simulink model "wiper_system"  (R2022b)
settings: Solver=VariableStepAuto  StartTime=0.0  StopTime=10  MaxStep=1e-3  RelTol=1e-3
undefined symbols (not defined in the file or in its folder): wiper_mode
settings Model: Creator=Dell  LastModifiedBy=Dell
settings DataIOCC: ExternalInput=[t, in1,in2]  SaveFormat=Array
settings DebuggingCC: ParameterPrecisionLossMsg=none

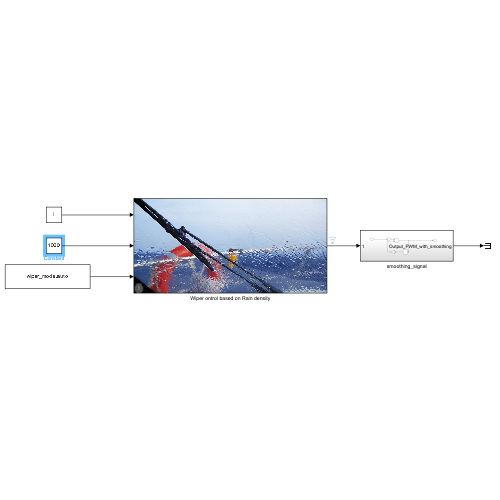
[thumbnail: Simulink's stored preview of the top-level diagram]
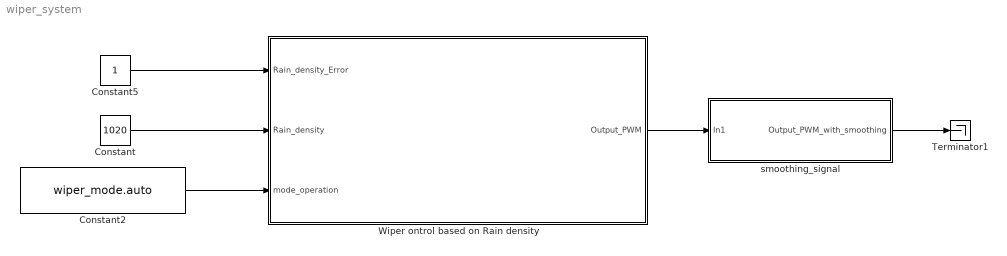
== system wiper_system ==
  Constant : Constant  Value=1020
  Constant2 : Constant  Value=wiper_mode.auto  OutDataTypeStr=Enum: wiper_mode
  Constant5 : Constant
  Terminator1 : Terminator
  Wiper ontrol based on Rain density : Subsystem
      mask Display: image('wiper.jpg');
  smoothing_signal : Subsystem
  wires:
  Constant5/1 -> Wiper ontrol based on Rain density/1(Rain_density_Error)
  Constant/1 -> Wiper ontrol based on Rain density/2(Rain_density)
  Constant2/1 -> Wiper ontrol based on Rain density/3(mode_operation)
  Wiper ontrol based on Rain density/1(Output_PWM) -> smoothing_signal/1(In1)
  smoothing_signal/1(Output_PWM_with_smoothing) -> Terminator1/1

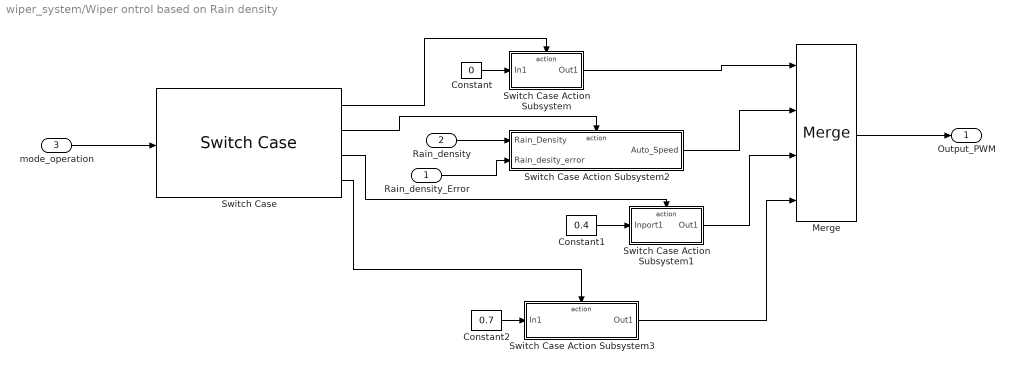
== system wiper_system/Wiper ontrol based on Rain density ==
  Rain_density_Error : Inport
  Rain_density : Inport  Port=2
  mode_operation : Inport  Port=3
  Constant : Constant  Value=0
  Constant1 : Constant  Value=0.4
  Constant2 : Constant  Value=0.7
  Merge : Merge  Inputs=4
  Switch Case : SwitchCase  CaseConditions=[wiper_mode.off,wiper_mode.auto,wiper_mode.low_speed,wiper_mode.high_speed]  ShowDefaultCase=off
  Switch Case Action Subsystem : Subsystem  TreatAsAtomicUnit=on
  Switch Case Action Subsystem1 : Subsystem  TreatAsAtomicUnit=on
  Switch Case Action Subsystem2 : Subsystem  TreatAsAtomicUnit=on
  Switch Case Action Subsystem3 : Subsystem  TreatAsAtomicUnit=on
  Output_PWM : Outport
  wires:
  Switch Case/1 -> Switch Case Action Subsystem/Action
  Switch Case/2 -> Switch Case Action Subsystem2/Action
  Switch Case/3 -> Switch Case Action Subsystem1/Action
  Switch Case/4 -> Switch Case Action Subsystem3/Action
  Constant2/1 -> Switch Case Action Subsystem3/1(In1)
  Constant1/1 -> Switch Case Action Subsystem1/1(Inport1)
  Constant/1 -> Switch Case Action Subsystem/1(In1)
  Rain_density_Error/1 -> Switch Case Action Subsystem2/2(Rain_desity_error)
  Switch Case Action Subsystem1/1(Out1) -> Merge/3
  Switch Case Action Subsystem3/1(Out1) -> Merge/4
  Rain_density/1 -> Switch Case Action Subsystem2/1(Rain_Density)
  Merge/1 -> Output_PWM/1
  Switch Case Action Subsystem/1(Out1) -> Merge/1
  Switch Case Action Subsystem2/1(Auto_Speed) -> Merge/2
  mode_operation/1 -> Switch Case/1

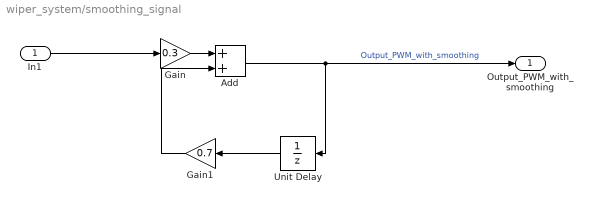
== system wiper_system/smoothing_signal ==
  In1 : Inport
  Add : Sum
  Gain : Gain  Gain=0.3
  Gain1 : Gain  Gain=0.7
  Unit Delay : UnitDelay  SampleTime=-1  HasFrameUpgradeWarning=on
  Output_PWM_with_smoothing : Outport
  wires:
  Add/1 -> Output_PWM_with_smoothing/1, Unit Delay/1  "Output_PWM_with_smoothing"
  Unit Delay/1 -> Gain1/1
  Gain1/1 -> Add/2
  Gain/1 -> Add/1
  In1/1 -> Gain/1

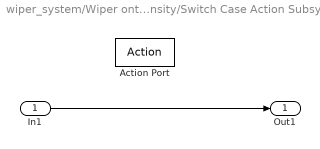
== system wiper_system/Wiper ontrol based on Rain density/Switch Case Action Subsystem ==
  In1 : Inport
  Action Port : ActionPort  ActionPortLabel=case [ off ]:
  Out1 : Outport
  wires:
  In1/1 -> Out1/1

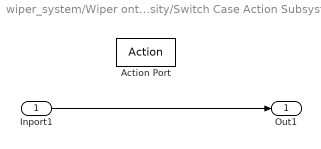
== system wiper_system/Wiper ontrol based on Rain density/Switch Case Action Subsystem1 ==
  Inport1 : Inport
  Action Port : ActionPort  ActionPortLabel=case [ low_speed ]:
  Out1 : Outport
  wires:
  Inport1/1 -> Out1/1

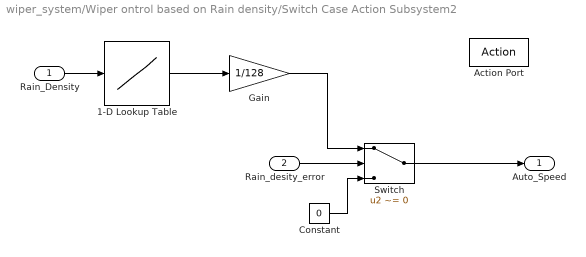
== system wiper_system/Wiper ontrol based on Rain density/Switch Case Action Subsystem2 ==
  Rain_Density : Inport
  Rain_desity_error : Inport  Port=2
  Action Port : ActionPort  ActionPortLabel=case [ auto ]:
  1-D Lookup Table : Lookup_n-D  NumberOfTableDimensions=1  LookupTableObject=''  BreakpointsForDimension1=[0 64 128 192 256]  BreakpointsForDimension1FirstPoint=10  BreakpointsForDimension2FirstPoint=10  BreakpointsForDimension1Spacing=12  BreakpointsForDimension2Spacing=12  IndexSearchMethod=Evenly spaced points  Table=[0 256 512 768 1023]  InternalRulePriority=Speed  RndMeth=Simplest
  Constant : Constant  Value=0
  Gain : Gain  Gain=1/128
  Switch : Switch  Criteria=u2 ~= 0  SaturateOnIntegerOverflow=off  InputSameDT=off
  Auto_Speed : Outport
  wires:
  Rain_desity_error/1 -> Switch/2
  Rain_Density/1 -> 1-D Lookup Table/1
  1-D Lookup Table/1 -> Gain/1
  Switch/1 -> Auto_Speed/1
  Constant/1 -> Switch/3
  Gain/1 -> Switch/1

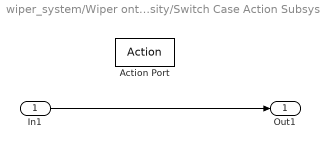
== system wiper_system/Wiper ontrol based on Rain density/Switch Case Action Subsystem3 ==
  In1 : Inport
  Action Port : ActionPort  ActionPortLabel=case [ high_speed ]:
  Out1 : Outport
  wires:
  In1/1 -> Out1/1
